simulink model "PIDsimulink"  (R2015a)
settings: Solver=ode45  StartTime=0.0  StopTime=10.0  RelTol=1e-3
values from neighbouring files (symbols this model uses):
  b = 0.1    [SilnikDC.m]    (also in algorytmgrzalka.m = [500;500;500]; funkcja.m; modelmplik.m)
  J = 0.01    [SilnikDC.m]    (also in funkcja.m; modelmplik.m; wirnik.m = 0.1; wirnik1.m = 0.1)
  K = 0.01    [SilnikDC.m]    (also in funkcja.m; modelmplik.m)
  Kd = 20    [SilnikDC.m]    (also in funkcja.m = pid(2); funkcja1.m = pid(3); grzalka.m = output(3); grzałka.m = output(3))
  Ki = 200    [SilnikDC.m]    (also in funkcja.m = pid(3); funkcja1.m = pid(2); grzalka.m = output(2); grzałka.m = output(2))
  Kp = 100    [SilnikDC.m]    (also in funkcja.m = pid(1); funkcja1.m = pid(1); grzalka.m = output(1); grzałka.m = output(1))
  L = 0.5    [SilnikDC.m]    (also in funkcja.m; modelmplik.m)
  R = 1    [SilnikDC.m]    (also in funkcja.m; modelmplik.m)
settings Model: Creator=Dawid  LastModifiedBy=Dawid

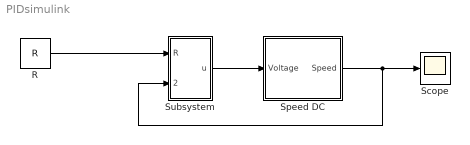
== system PIDsimulink ==
  R : Constant  Value=R
  Scope : Scope
  Speed DC : Subsystem
  Subsystem : Subsystem
  wires:
  Speed DC/1("Speed ") -> Scope/1, Subsystem/2(speed)
  R/1 -> Subsystem/1("R ")
  Subsystem/1(u) -> Speed DC/1(Voltage)

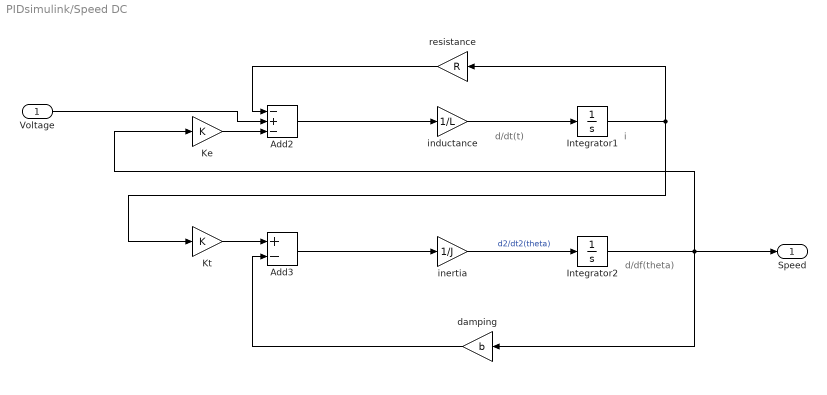
== system PIDsimulink/Speed DC ==
  note: i
  note: d/dt(t)
  note: d/df(theta)
  Voltage : Inport
  " damping" : Gain  Gain=b
  Add2 : Sum  Inputs=-+-
  Add3 : Sum  Inputs=+-
  Integrator1 : Integrator
  Integrator2 : Integrator
  "Ke " : Gain  Gain=K
  Kt : Gain  Gain=K
  inductance : Gain  Gain=1/L
  inertia : Gain  Gain=1/J
  resistance : Gain  Gain=R
  "Speed " : Outport
  wires:
  Voltage/1 -> Add2/2
  resistance/1 -> Add2/1
  Integrator2/1 -> "Ke "/1, " damping"/1, "Speed "/1
  inductance/1 -> Integrator1/1
  inertia/1 -> Integrator2/1  "d2/dt2(theta)"
  " damping"/1 -> Add3/2
  Kt/1 -> Add3/1
  "Ke "/1 -> Add2/3
  Add3/1 -> inertia/1
  Add2/1 -> inductance/1
  Integrator1/1 -> Kt/1, resistance/1

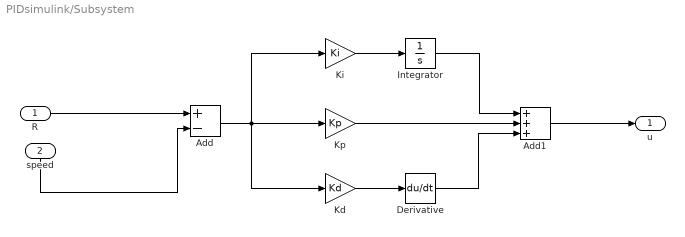
== system PIDsimulink/Subsystem ==
  "R " : Inport
  speed : Inport  Port=2
  Add : Sum  Inputs=+-
  Add1 : Sum  Inputs=+++
  Derivative : Derivative
  Integrator : Integrator
  Kd : Gain  Gain=Kd
  "Ki " : Gain  Gain=Ki
  Kp : Gain  Gain=Kp
  u : Outport
  wires:
  Kp/1 -> Add1/2
  Integrator/1 -> Add1/1
  Kd/1 -> Derivative/1
  "Ki "/1 -> Integrator/1
  Add/1 -> Kd/1, "Ki "/1, Kp/1
  Add1/1 -> u/1
  Derivative/1 -> Add1/3
  "R "/1 -> Add/1
  speed/1 -> Add/2
